simulink model "zouzhihua"  (R2018b)
settings: Solver=ode4  StartTime=0.0  StopTime=10  FixedStep=0.001  RelTol=1e-3  EnableMultiTasking=on
settings Model: ExtModeTrigMode=oneshot  ExtModeArmWhenConnect=off  Creator=hp  LastModifiedBy=Administrator
settings DataIOCC: SaveFormat=Array  SignalLoggingSaveFormat=ModelDataLogs  SignalLoggingName=sigsOut
settings OptimizationCC: BooleanDataType=off  ExpressionDepthLimit=2147483647  InitFltsAndDblsToZero=on  LifeSpan=inf
settings DebuggingCC: SaveWithParameterizedLinksMsg=none  UnderspecifiedInitializationDetection=Classic  MergeDetectMultiDrivingBlocksExec=none  SignalResolutionControl=TryResolveAllWithWarning  MultiTaskDSMMsg=warning  MultiTaskCondExecSysMsg=none  FcnCallInpInsideContextMsg=warning  StateNameClashWarn=warning  SFUnexpectedBacktrackingDiag=warning  SFNoUnconditionalDefaultTransitionDiag=warning  SFExecutionAtInitializationDiag=none
settings HardwareCC: ProdBitPerPointer=32  ProdBitPerSizeT=32  ProdBitPerPtrDiffT=32  ProdLargestAtomicFloat=None  ProdIntDivRoundTo=Undefined  ProdEndianess=Unspecified  ProdWordSize=32  ProdHWDeviceType=32-bit Generic  TargetUnknown=on
settings ModelReferenceCC: PropagateSignalLabelsOutOfModel=off
settings SFSimCC: SimUseLocalCustomCode=off
settings RTWCC: RTWUseLocalCustomCode=off
settings CodeAppCC: StateflowObjectComments=on
settings GRTTargetCC: TargetFcnLib=ansi_tfl_tmw.mat  TargetLangStandard=C89/C90 (ANSI)  GeneratePreprocessorConditionals=Disable all  CombineOutputUpdateFcns=off  GRTInterface=on
settings ConfigComp: CovMetricSettings=dw  CovHtmlReporting=on  CovSaveCumulativeToWorkspaceVar=on  CovSaveSingleToWorkspaceVar=on  CovExternalEMLEnable=off

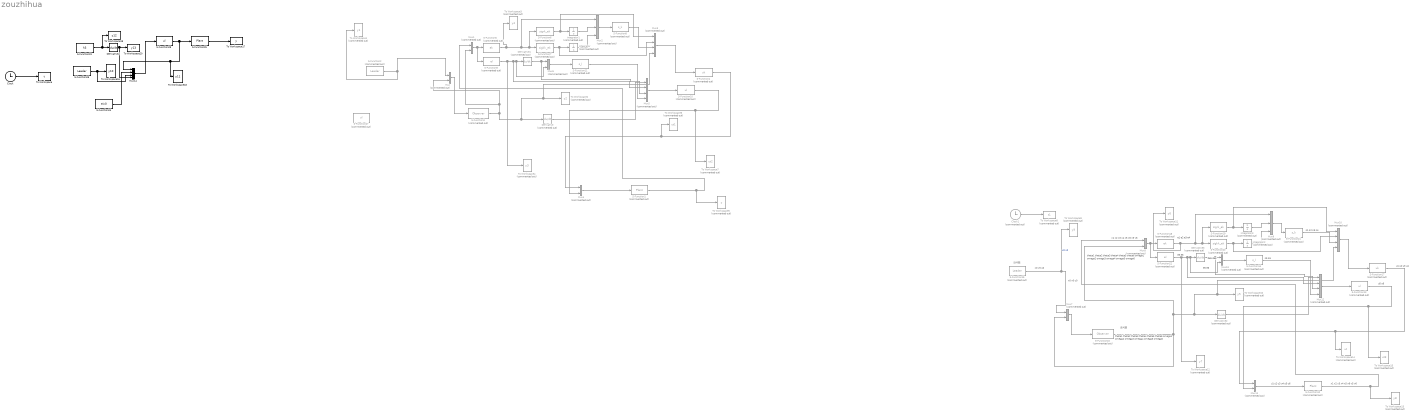
== system zouzhihua ==
  note: x0 v0 u0
  note: e5 e6
  note: x0 v0 u0
  note: u1 u2 u3 u4 u5 u6
  note: theta1 theta2 theta3 theta4 theta5 theta6
      | omega1 omega2 omega3 omega4 omega5 omega6
  note: e1 e2 e3 e4
  note: s5 s6
  note: x1 x2 x3 x4 x5 x6 v5 v6
  note: s1 s2 s3 s4
  note: u5 u6
  note: theta1 theta2 theta3 theta4 theta5 theta6
      | omega1 omega2 omega3 omega4 omega5 omega6
  note: 没问题
  note: x1 x2 x3 x4 x5 x6 v5 v6
  note: 没问题
  note: u1 u2 u3 u4
  note: e5 e6
  note: de5 de6
  Clock : Clock
  Clock1 : Clock  Commented=on
  Derivative{,1..3} (4 alike) : Derivative  Commented=on
  Derivative4 : Derivative
  Integrator{,1..3} (4 alike) : Integrator  Commented=on
  Mux{,1,4,6..8,11,13} (8 alike) : Mux  Commented=on  Inputs=2
  Mux{3,5,10,12} (4 alike) : Mux  Commented=on
  Mux14 : Mux
  Mux2 : Mux  Commented=on  Inputs=3
  Mux9 : Mux  Commented=on  Inputs=3
  S-Function1 : S-Function  Commented=on  FunctionName=Plant  SFunctionDeploymentMode=off  EnableBusSupport=off
  S-Function10 : S-Function  Commented=on  FunctionName=ul  SFunctionDeploymentMode=off  EnableBusSupport=off
  S-Function11 : S-Function  Commented=on  FunctionName=s_l  SFunctionDeploymentMode=off  EnableBusSupport=off
  S-Function12 : S-Function  Commented=on  FunctionName=Plant  SFunctionDeploymentMode=off  EnableBusSupport=off
  S-Function13 : S-Function  Commented=on  FunctionName=ul  SFunctionDeploymentMode=off  EnableBusSupport=off
  S-Function14 : S-Function  Commented=on  FunctionName=s_l  SFunctionDeploymentMode=off  EnableBusSupport=off
  S-Function15 : S-Function  Commented=on  FunctionName=Leader  SFunctionDeploymentMode=off  EnableBusSupport=off
  S-Function16 : S-Function  Commented=on  FunctionName=Observer  SFunctionDeploymentMode=off  EnableBusSupport=off
  S-Function17 : S-Function  Commented=on  FunctionName=uk  SFunctionDeploymentMode=off  EnableBusSupport=off
  S-Function18 : S-Function  Commented=on  FunctionName=ek  SFunctionDeploymentMode=off  EnableBusSupport=off
  S-Function19 : S-Function  Commented=on  FunctionName=sigrk_ek  SFunctionDeploymentMode=off  EnableBusSupport=off
  S-Function2 : S-Function  Commented=on  FunctionName=Leader  SFunctionDeploymentMode=off  EnableBusSupport=off
  S-Function20 : S-Function  Commented=on  FunctionName=sigkk_ek  SFunctionDeploymentMode=off  EnableBusSupport=off
  S-Function21 : S-Function  Commented=on  FunctionName=s_k  SFunctionDeploymentMode=off  EnableBusSupport=off
  S-Function22 : S-Function  Commented=on  FunctionName=el  SFunctionDeploymentMode=off  EnableBusSupport=off
  S-Function23 : S-Function  FunctionName=h3  SFunctionDeploymentMode=off  EnableBusSupport=off
  S-Function24 : S-Function  FunctionName=eix0  SFunctionDeploymentMode=off  EnableBusSupport=off
  S-Function25 : S-Function  FunctionName=Plant  SFunctionDeploymentMode=off  EnableBusSupport=off
  S-Function26 : S-Function  FunctionName=Leader  SFunctionDeploymentMode=off  EnableBusSupport=off
  S-Function27 : S-Function  Commented=on  FunctionName=ul  SFunctionDeploymentMode=off  EnableBusSupport=off
  S-Function28 : S-Function  FunctionName=ul  SFunctionDeploymentMode=off  EnableBusSupport=off
  S-Function3 : S-Function  Commented=on  FunctionName=Observer  SFunctionDeploymentMode=off  EnableBusSupport=off
  S-Function4 : S-Function  Commented=on  FunctionName=uk  SFunctionDeploymentMode=off  EnableBusSupport=off
  S-Function5 : S-Function  Commented=on  FunctionName=ek  SFunctionDeploymentMode=off  EnableBusSupport=off
  S-Function6 : S-Function  Commented=on  FunctionName=sigrk_ek  SFunctionDeploymentMode=off  EnableBusSupport=off
  S-Function7 : S-Function  Commented=on  FunctionName=sigkk_ek  SFunctionDeploymentMode=off  EnableBusSupport=off
  S-Function8 : S-Function  Commented=on  FunctionName=s_k  SFunctionDeploymentMode=off  EnableBusSupport=off
  S-Function9 : S-Function  Commented=on  FunctionName=el  SFunctionDeploymentMode=off  EnableBusSupport=off
  To Workspace : ToWorkspace  VariableName=t  SampleTime=-1
  To Workspace1 : ToWorkspace  Commented=on  VariableName=y1  SampleTime=-1
  To Workspace10 : ToWorkspace  Commented=on  VariableName=y5  SampleTime=-1
  To Workspace11 : ToWorkspace  Commented=on  VariableName=y6  SampleTime=-1
  To Workspace12 : ToWorkspace  Commented=on  VariableName=y7  SampleTime=-1
  To Workspace13 : ToWorkspace  Commented=on  VariableName=y8  SampleTime=-1
  To Workspace14 : ToWorkspace  Commented=on  VariableName=ut  SampleTime=-1
  To Workspace15 : ToWorkspace  Commented=on  VariableName=ut3  SampleTime=-1
  To Workspace16 : ToWorkspace  VariableName=y10  SampleTime=-1
  To Workspace17 : ToWorkspace  VariableName=y  SampleTime=-1
  To Workspace18 : ToWorkspace  VariableName=y11  SampleTime=-1
  To Workspace19 : ToWorkspace  VariableName=y12  SampleTime=-1
  To Workspace2 : ToWorkspace  Commented=on  VariableName=y2  SampleTime=-1
  To Workspace20 : ToWorkspace  VariableName=y13  SampleTime=-1
  To Workspace3 : ToWorkspace  Commented=on  VariableName=y4  SampleTime=-1
  To Workspace4 : ToWorkspace  Commented=on  VariableName=y3  SampleTime=-1
  To Workspace5 : ToWorkspace  Commented=on  VariableName=y  SampleTime=-1
  To Workspace6 : ToWorkspace  Commented=on  VariableName=ut1  SampleTime=-1
  To Workspace7 : ToWorkspace  Commented=on  VariableName=ut2  SampleTime=-1
  To Workspace8 : ToWorkspace  Commented=on  VariableName=t1  SampleTime=-1
  To Workspace9 : ToWorkspace  Commented=on  VariableName=y9  SampleTime=-1
  wires:
  Clock/1 -> To Workspace/1
  S-Function2/1 -> To Workspace1/1, Mux/1
  Mux/1 -> S-Function3/1
  S-Function3/1 -> Mux/2, Mux1/2, Mux3/4, To Workspace2/1, Derivative/1
  Mux1/1 -> S-Function9/1, S-Function5/1
  S-Function1/1 -> To Workspace5/1, Mux1/1
  S-Function5/1 -> To Workspace3/1, Mux2/1, S-Function7/1, S-Function6/1
  S-Function7/1 -> Mux3/2, Integrator/1
  S-Function6/1 -> Mux3/1, Integrator1/1
  Mux2/1 -> S-Function8/1
  Integrator1/1 -> Mux2/2
  S-Function8/1 -> Mux3/3
  Mux3/1 -> S-Function4/1
  Mux4/1 -> S-Function1/1
  S-Function4/1 -> To Workspace6/1, Mux4/1
  S-Function10/1 -> To Workspace7/1, Mux4/2
  S-Function9/1 -> To Workspace4/1, Mux5/2, Mux6/2, Derivative1/1
  Derivative1/1 -> Mux6/1, Mux5/3
  Mux6/1 -> S-Function11/1
  Derivative/1 -> Mux5/1
  S-Function11/1 -> Mux5/4
  Mux5/1 -> S-Function10/1
  Integrator/1 -> Mux2/3
  Integrator2/1 -> Mux9/3
  S-Function16/1 -> Mux10/4, To Workspace10/1, Derivative2/1, Mux8/2, Mux7/2
  S-Function12/1 -> To Workspace13/1, Mux8/1
  S-Function13/1 -> To Workspace15/1, Mux11/2
  Mux12/1 -> S-Function13/1
  Mux11/1 -> S-Function12/1
  S-Function20/1 -> Mux10/2, Integrator2/1
  S-Function14/1 -> Mux12/4
  S-Function15/1 -> Mux7/1, To Workspace9/1  "x0 v0"
  S-Function22/1 -> To Workspace12/1, Mux12/2, Mux13/2, Derivative3/1
  Derivative2/1 -> Mux12/1
  Integrator3/1 -> Mux9/2
  S-Function21/1 -> Mux10/3
  Mux7/1 -> S-Function16/1
  S-Function19/1 -> Mux10/1, Integrator3/1
  Mux13/1 -> S-Function14/1
  S-Function17/1 -> To Workspace14/1, Mux11/1
  Derivative3/1 -> Mux13/1, Mux12/3
  S-Function18/1 -> To Workspace11/1, Mux9/1, S-Function20/1, S-Function19/1
  Mux10/1 -> S-Function17/1
  Mux8/1 -> S-Function22/1, S-Function18/1
  Mux9/1 -> S-Function21/1
  Clock1/1 -> To Workspace8/1
  S-Function26/1 -> Mux14/3, To Workspace16/1
  S-Function24/1 -> Mux14/2
  S-Function23/1 -> To Workspace19/1, Derivative4/1
  Derivative4/1 -> To Workspace20/1, Mux14/4
  Mux14/1 -> S-Function28/1
  S-Function25/1 -> To Workspace17/1
  S-Function28/1 -> To Workspace18/1, Mux14/1, S-Function25/1
